simulink model "closedloop_model_nolimit"  (R2024a)
settings: Solver=VariableStepAuto  StartTime=0.0  StopTime=20  RelTol=1e-3
undefined symbols (not defined in the file): Kp, Td, Ti
libraries: cstblocks x2
settings Model: SimulationMode=accelerator  Creator=thoma  LastModifiedBy=thoma

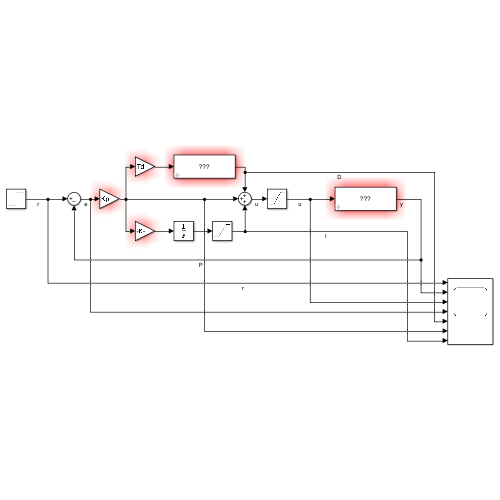
[thumbnail: Simulink's stored preview of the top-level diagram]
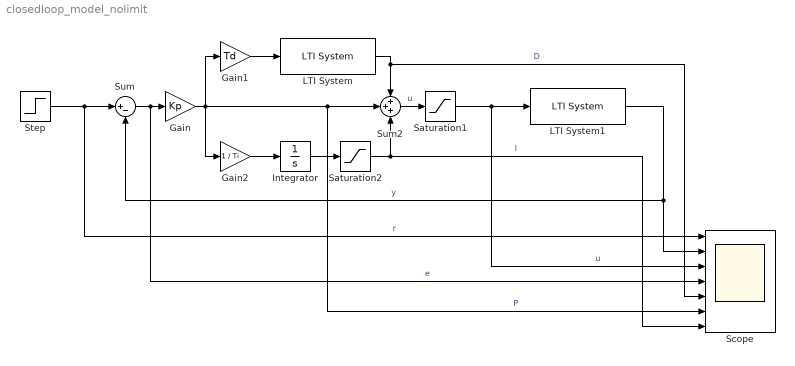
== system closedloop_model_nolimit ==
  Gain : Gain  Gain=Kp
  Gain1 : Gain  Gain=Td
  Gain2 : Gain  Gain=1 / Ti
  Integrator : Integrator
  LTI System : cstblocks/LTI System  sys=F  IC=[]  PadeOrder=0
  LTI System1 : cstblocks/LTI System  sys=G  IC=[]  PadeOrder=0
  Saturation1 : Saturate  UpperLimit=5  LowerLimit=-5
  Saturation2 : Saturate  UpperLimit=5  LowerLimit=-5
  Scope : Scope  NumInputPorts=7
  Step : Step  Time=0  SampleTime=0
  Sum : Sum  Inputs=|+-
  Sum2 : Sum  Inputs=+++
  wires:
  Gain/1 -> Gain2/1, Scope/6, Sum2/2, Gain1/1  "P"
  Step/1 -> Sum/1, Scope/1  "r"
  Gain1/1 -> LTI System/1
  Gain2/1 -> Integrator/1
  LTI System/1 -> Sum2/1, Scope/5  "D"
  LTI System1/1 -> Sum/2, Scope/2  "y"
  Integrator/1 -> Saturation2/1
  Sum2/1 -> Saturation1/1  "u"
  Saturation1/1 -> Scope/3, LTI System1/1  "u"
  Saturation2/1 -> Scope/7, Sum2/3  "I"
  Sum/1 -> Scope/4, Gain/1  "e"
